simulink library "Is_equal_scalar"  (Simulink 8.1)
settings: Solver=ode45  StartTime=0.0  StopTime=10.0  RelTol=1e-3
libraries: simulink x1
settings Model: Creator=dejanira  LastModifiedBy=dejanira

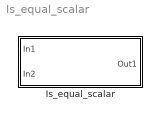
== system Is_equal_scalar ==
  Is_equal_scalar : Subsystem  TreatAsAtomicUnit=on  mask(Is_equal_scalar){}
      mask Display:
      | port_label('input',1,'v1')
      | port_label('input',2,'v2')
      | port_label('output',1,'T/F')

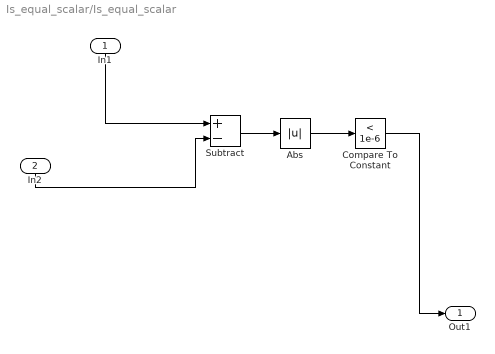
== system Is_equal_scalar/Is_equal_scalar ==
  In1 : Inport
  In2 : Inport  Port=2
  Abs : Abs
  Compare To Constant : simulink/Logic and Bit Operations/Compare To Constant  relop=<  const=1e-6  OutDataTypeStr=boolean
  Subtract : Sum  Inputs=+-
  Out1 : Outport
  wires:
  In1/1 -> Subtract/1
  In2/1 -> Subtract/2
  Subtract/1 -> Abs/1
  Abs/1 -> Compare To Constant/1
  Compare To Constant/1 -> Out1/1
